simulink model "generateDuty"  (R2024b)
settings: Solver=FixedStepAuto  StartTime=0.0  StopTime=10.0  FixedStep=0.0001  RelTol=1e-3
settings Model: Creator=sung0058  LastModifiedBy=tnoguchi
settings DataIOCC: SaveOutput=off  SaveTime=off
settings OptimizationCC: DefaultParameterBehavior=Inlined  EnhancedBackFolding=on  PassReuseOutputArgsAs=Individual arguments  ZeroExternalMemoryAtStartup=off  ZeroInternalMemoryAtStartup=off  OptimizeBlockOrder=speed  DifferentSizesBufferReuse=on  OptimizationCustomize=off  EfficientTunableParamExpr=on
settings DebuggingCC: ParameterTunabilityLossMsg=error
settings SFSimCC: MATLABDynamicMemAlloc=off
settings RTWCC: Description=Embedded Coder  SystemTargetFile=ert.tlc  GenCodeOnly=on  TemplateMakefile=ert_default_tmf
settings CodeAppCC: ForceParamTrailComments=on  IgnoreCustomStorageClasses=off  OperatorAnnotations=on  SimulinkDataObjDesc=on  SFDataObjDesc=on  InsertBlockDesc=on
settings ERTTargetCC: TargetLangStandard=C99 (ISO)  ERTCustomFileTemplate=example_file_process.tlc
settings ConfigComp: CovBoundaryAbsTol=1.0e-5

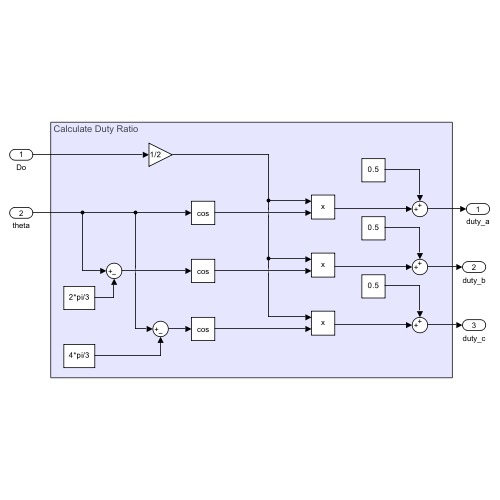
[thumbnail: Simulink's stored preview of the top-level diagram]
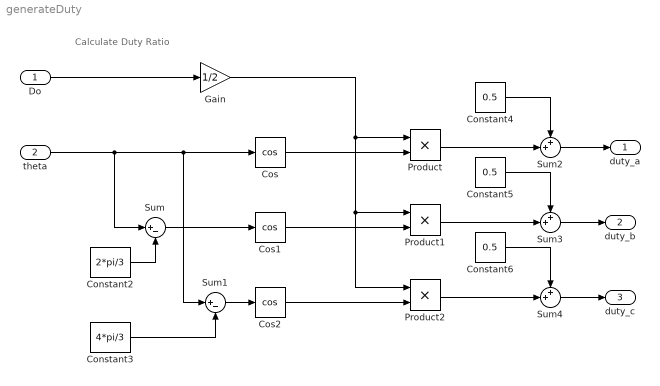
== system generateDuty ==
  note: Calculate Duty Ratio
  Do : Inport  OutDataTypeStr=double  PortDimensions=1  SampleTime=[0.0001,0]
  theta : Inport  Port=2  OutDataTypeStr=double  PortDimensions=1  SampleTime=[0.0001,0]
  Constant2 : Constant  Value=2*pi/3
  Constant3 : Constant  Value=4*pi/3
  Constant4 : Constant  Value=0.5
  Constant5 : Constant  Value=0.5
  Constant6 : Constant  Value=0.5
  Cos : Trigonometry  Operator=cos
  Cos1 : Trigonometry  Operator=cos
  Cos2 : Trigonometry  Operator=cos
  Gain : Gain  Gain=1/2
  Product : Product
  Product1 : Product
  Product2 : Product
  Sum : Sum  Inputs=|+-
  Sum1 : Sum  Inputs=|+-
  Sum2 : Sum  Inputs=++|
  Sum3 : Sum  Inputs=++|
  Sum4 : Sum  Inputs=++|
  duty_a : Outport  OutDataTypeStr=double  PortDimensions=1  SampleTime=[0.0001,0]
  duty_b : Outport  Port=2  OutDataTypeStr=double  PortDimensions=1  SampleTime=[0.0001,0]
  duty_c : Outport  Port=3  OutDataTypeStr=double  PortDimensions=1  SampleTime=[0.0001,0]
  wires:
  Gain/1 -> Product1/1, Product2/1, Product/1
  Cos2/1 -> Product2/2
  Constant6/1 -> Sum4/1
  Do/1 -> Gain/1
  Constant5/1 -> Sum3/1
  Constant3/1 -> Sum1/2
  Product1/1 -> Sum3/2
  Cos1/1 -> Product1/2
  Cos/1 -> Product/2
  Sum1/1 -> Cos2/1
  Product/1 -> Sum2/2
  Sum4/1 -> duty_c/1
  Sum2/1 -> duty_a/1
  Constant4/1 -> Sum2/1
  Sum3/1 -> duty_b/1
  theta/1 -> Sum1/1, Cos/1, Sum/1
  Sum/1 -> Cos1/1
  Product2/1 -> Sum4/2
  Constant2/1 -> Sum/2
